simulink model "uGrid_1PH_hd_ATD2"  (R2018a)
settings: Solver=VariableStepAuto  StartTime=0.0  StopTime=0.8  FixedStep=1e-6  MaxStep=1e-4  RelTol=1e-3
PreLoadFcn:
  | SimulinkInit
InitFcn:
  | SimulinkInit
StopFcn:
  | EndingScript
values from neighbouring files (symbols this model uses):
  Ad = sysd.A    [SimulinkInit.m]
  Bd = sysd.B    [SimulinkInit.m]
  C1 = Cd(2,:)    [SimulinkInit.m]
  C10 = Cd(1,:)    [SimulinkInit.m]
  C11 = Cd(2,:)    [SimulinkInit.m]
  C12 = Cd(3,:)    [SimulinkInit.m]
  C2 = Cd(3,:)    [SimulinkInit.m]
  C3 = Cd(4,:)    [SimulinkInit.m]
  C4 = Cd(1,:)    [SimulinkInit.m]
  C5 = Cd(3,:)    [SimulinkInit.m]
  C6 = Cd(4,:)    [SimulinkInit.m]
  C7 = Cd(1,:)    [SimulinkInit.m]
  C8 = Cd(2,:)    [SimulinkInit.m]
  C9 = Cd(4,:)    [SimulinkInit.m]
  Cd = sysd.C    [SimulinkInit.m]
  T1 = 0.4    [parametros_BIO.m]
  T2 = 1    [parametros_BIO.m]
  T3 = 15    [parametros_BIO.m]
  T4 = 2.5    [parametros_BIO.m]
  T5 = 3.3    [parametros_BIO.m]
  Tao1 = 0.5    [SimulinkInit.m]
  tm = 1e-4    (= 0.0001)    [SimulinkInit.m]
undefined symbols (not defined in the file or in its folder): F1, F10, F11, F12, F2, F3, F4, F5, F6, F7, F8, F9, G, GF, H1, H10, H11, H12, H2, H3, H4, H5, H6, H7, H8, H9, Ion, K10U, K11U, K12U, K1U, K2U, K3U, K4U, K5U, K6U, K7U, K8U, K9U, Lithium, ss1, ss2, T10, T11, T12, T6, T7, T8, T9
libraries: powerlib x59, dsparch4 x17, truetime x12, powerlib_meascontrol x6, simulink x2, dspstat3 x2, dspfdesign x1, electricdrivelib x1
(part 1 of 3)
settings Model: Creator=erich  LastModifiedBy=cmparedes
settings CodeAppCC: StateflowObjectComments=on
settings SimscapeCC: SimscapeNormalizeSystem=off

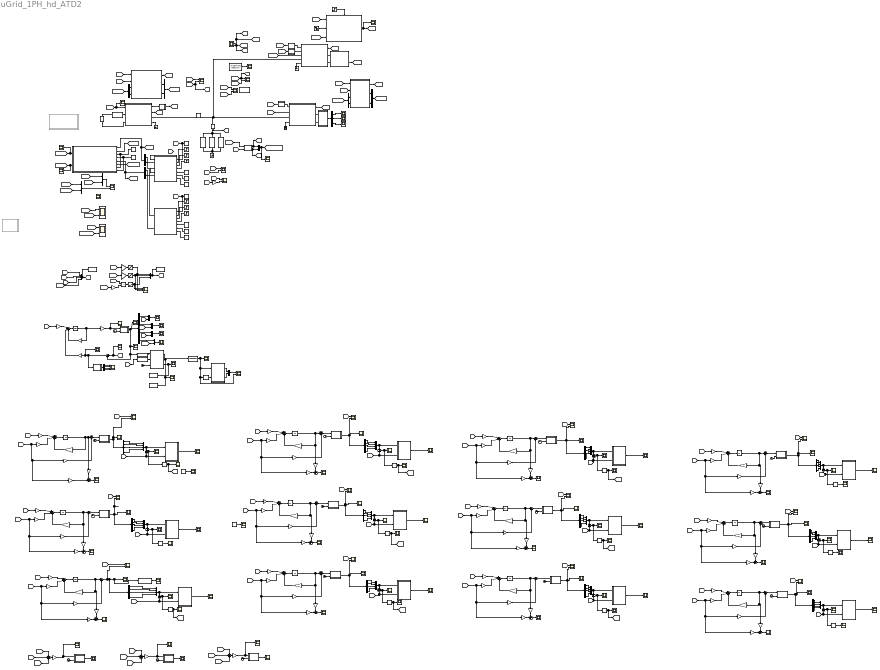
== system uGrid_1PH_hd_ATD2 ==
  note: DIESEL VSI
  note: Load
  note: BIO - CSI
  note: RENEWABLE - CSI
  note: Nodo De Optimizacion
  1Ph_Inverter_bio : Subsystem  mask{st_time=0, f_sw=12000, samp_f=1e-6}
      mask prompts: st_time "Tiempo muerto (Start)"; f_sw "Switching frequency"; samp_f "samplig"
      mask Display:
      | port_label('input', 1, 'd', 'texmode', 'on')
      | 
      | port_label('lconn', 1, 'DC +')
      | port_label('lconn', 2, 'DC -')
      | 
      | 
      | port_label('rconn', 1, 'V_{out+}')
      | port_label('rconn', 2, 'B_{out-}')
      | 
      | 
      | port_label('output', 1, 'I_{out}', 'texmode', 'on')
      | port_label('output', 2, 'V_{out}', 'texmode', 'on')
      | 
      | plot([0.1 .9], [0.1 .9])
      | plot([0.2 .4], [.7 .7])
      | plot([0.2 .24], [.65 .65])
      | plot([0.28 .32], [.65 .65])
      | plot([0.36 .40], [.65 .65])
      | 
      | plot([.5:.01:.7], .25+sin(30*[.2:.01:.4])/10)
  1Ph_Inverter_bio1 : Subsystem  mask{st_time=0, f_sw=12000, samp_f=1e-6}
      mask prompts: st_time "Tiempo muerto (Start)"; f_sw "Switching frequency"; samp_f "samplig"
      mask Display:
      | port_label('input', 1, 'd', 'texmode', 'on')
      | 
      | port_label('lconn', 1, 'DC +')
      | port_label('lconn', 2, 'DC -')
      | 
      | 
      | port_label('rconn', 1, 'V_{out+}')
      | port_label('rconn', 2, 'B_{out-}')
      | 
      | 
      | port_label('output', 1, 'I_{out}', 'texmode', 'on')
      | port_label('output', 2, 'V_{out}', 'texmode', 'on')
      | port_label('output', 3, 'I_{cap}', 'texmode', 'on')
      | 
      | plot([0.1 .9], [0.1 .9])
      | plot([0.2 .4], [.7 .7])
      | plot([0.2 .24], [.65 .65])
      | plot([0.28 .32], [.65 .65])
      | plot([0.36 .40], [.65 .65])
      | 
      | plot([.5:.01:.7], .25+sin(30*[.2:.01:.4])/10)
  1Ph_Inverter_diesel : Subsystem  mask{st_time=0, f_sw=12000, samp_f=1e-6}
      mask prompts: st_time "Tiempo muerto (Start)"; f_sw "Switching frequency"; samp_f "Sampling frequency"
      mask Display:
      | port_label('input', 1, 'd', 'texmode', 'on')
      | 
      | port_label('lconn', 1, 'DC +')
      | port_label('lconn', 2, 'DC -')
      | 
      | 
      | port_label('rconn', 1, 'V_{out+}')
      | port_label('rconn', 2, 'B_{out-}')
      | 
      | 
      | port_label('output', 1, 'I_{out}', 'texmode', 'on')
      | port_label('output', 2, 'V_{out}', 'texmode', 'on')
      | 
      | plot([0.1 .9], [0.1 .9])
      | plot([0.2 .4], [.7 .7])
      | plot([0.2 .24], [.65 .65])
      | plot([0.28 .32], [.65 .65])
      | plot([0.36 .40], [.65 .65])
      | 
      | plot([.5:.01:.7], .25+sin(30*[.2:.01:.4])/10)
  BioMassGenerator : Subsystem  Commented=on
  Bus Selector : BusSelector  OutputSignals=SOC (%),Current (A),Voltage (V)
  CSI_Control_BIO : Subsystem
  CSI_Control_DIESEL : Subsystem
  Clock{,1,3..16} (16 alike) : Clock
  Constant : Constant  Value=1000
  Constant{1,4..5,7} (4 alike) : Constant  Value=4000
  Constant2 : Constant  Value=11210
  Constant3 : Constant  Value=5000
  Constant6 : Constant  Value=5000
  DC 1000V : powerlib/Electrical Sources/DC Voltage Source  Amplitude=1000  Measurements=None
  DIESEL + Rectifier System : Subsystem
  Delay2 : Delay  DelayLength=1
  Demux : Demux  Outputs=2
  Demux1 : Demux  Outputs=2
  Demux{3..14} (12 alike) : Demux  Outputs=5
  Demux19 : Demux
  Demux2 : Demux
  Derivative{,1..2,4..12} (12 alike) : Derivative  CoefficientInTFapproximation=0
  Derivative3 : Derivative
  DynMat : Constant  Value=G
  DynMat_RespLibre : Constant  Value=GF
  FRACASO : Subsystem  Commented=on
  Gain : Gain  Gain=1/3
  Gain1 : Gain  Gain=1/3
  Gain2 : Gain  Gain=-1
  Gain3 : Gain  Gain=1/3
  Gain4 : Gain  Gain=2000
  Gain5 : Gain  Gain=2
  Gain6 : Gain  Gain=2000
  Ground{,1..3} (4 alike) : powerlib/Elements/Ground  LConnTagsString=a
  Highpass Filter : dspfdesign/Highpass Filter  FilterType=FIR  DesignForMinimumOrder=on  FilterOrder=50  StopbandFrequency=50  PassbandFrequency=60  StopbandAttenuation=80  PassbandRipple=0.1  InheritSampleRate=off  SampleRate=1/tm  SimulateUsing=Interpreted execution  roundingMode=Floor  coeffsDataTypeStr=fixdt(1,16)
      settings: SourceProductName=DSP System Toolbox
  Hw5 : dsparch4/Analog Filter Design  method=Bessel  filttype=Lowpass  N=20  Wlo=60*2*pi  Whi=80  Rp=2  Rs=80
  I sens A : powerlib/Measurements/Current Measurement  PhasorSimulation=off  OutputType=Complex  PSBequivalent=0
  LinearProg : MATLAB Function  TreatAsAtomicUnit=on  SystemSampleTime=1e-3
  LinearProg1 : MATLAB Function  TreatAsAtomicUnit=on  SystemSampleTime=1e-3
  MATLAB Function : MATLAB Function  TreatAsAtomicUnit=on
  MATLAB Function1 : MATLAB Function  TreatAsAtomicUnit=on
  MATLAB Function12 : MATLAB Function  TreatAsAtomicUnit=on
  MATLAB Function13 : MATLAB Function  TreatAsAtomicUnit=on
  MATLAB Function15 : MATLAB Function  TreatAsAtomicUnit=on
  MATLAB Function16 : MATLAB Function  TreatAsAtomicUnit=on
  MATLAB Function17 : MATLAB Function  TreatAsAtomicUnit=on
  MATLAB Function18 : MATLAB Function  TreatAsAtomicUnit=on
  MATLAB Function19 : MATLAB Function  TreatAsAtomicUnit=on
  MATLAB Function2 : MATLAB Function  TreatAsAtomicUnit=on
  MATLAB Function20 : MATLAB Function  TreatAsAtomicUnit=on
  MATLAB Function21 : MATLAB Function  TreatAsAtomicUnit=on
  MATLAB Function22 : MATLAB Function  TreatAsAtomicUnit=on
  MATLAB Function24 : MATLAB Function  TreatAsAtomicUnit=on
  MATLAB Function25 : MATLAB Function  TreatAsAtomicUnit=on
  MATLAB Function26 : MATLAB Function  TreatAsAtomicUnit=on
  MATLAB Function27 : MATLAB Function  TreatAsAtomicUnit=on
  MATLAB Function28 : MATLAB Function  TreatAsAtomicUnit=on
  MATLAB Function29 : MATLAB Function  TreatAsAtomicUnit=on
  MATLAB Function3 : MATLAB Function  TreatAsAtomicUnit=on
  MATLAB Function30 : MATLAB Function  TreatAsAtomicUnit=on
  MATLAB Function31 : MATLAB Function  TreatAsAtomicUnit=on
  MATLAB Function32 : MATLAB Function  TreatAsAtomicUnit=on
  MATLAB Function33 : MATLAB Function  TreatAsAtomicUnit=on
  MATLAB Function34 : MATLAB Function  TreatAsAtomicUnit=on
  MATLAB Function35 : MATLAB Function  TreatAsAtomicUnit=on
  MATLAB Function37 : MATLAB Function  TreatAsAtomicUnit=on
  MATLAB Function7 : MATLAB Function  TreatAsAtomicUnit=on
  MATLAB Function8 : MATLAB Function  TreatAsAtomicUnit=on
  MATLAB Function9 : MATLAB Function  TreatAsAtomicUnit=on
  MPC Controller : Subsystem
  MeasureNode_I1 : Subsystem
  MeasureNode_I2 : Subsystem
  MeasureNode_I3 : Subsystem
  MeasureNode_I4 : Subsystem
  Mux{,1..6,9..12,14} (12 alike) : Mux  Inputs=2
  Mux{8,13,15..25} (13 alike) : Mux
  Mux7 : Mux  Inputs=3
  P_lp_bio : Constant  Value=500
  P_lp_diesel : Constant  Value=300
  Power : powerlib_meascontrol/Measurements/Power  Freq=60  Vinit=[1, 0]  Iinit=[1, 0]  Ts=0
      settings: SourceProductName=Simscape Power Systems
  Product1 : Product
  RL : powerlib/Elements/Series RLC Branch  LConnTagsString=__new0  RConnTagsString=__new0  BranchType=R  Resistance=10  Inductance=500e-3  SetiL0=off  InitialCurrent=0  Capacitance=100e-6  Setx0=off  InitialVoltage=0  Measurements=None
  RL1 : powerlib/Elements/Series RLC Branch  LConnTagsString=__new0  RConnTagsString=__new0  BranchType=RL  Resistance=10  Inductance=5.2  SetiL0=off  InitialCurrent=0  Capacitance=100e-6  Setx0=off  InitialVoltage=0  Measurements=None
  RL2 : powerlib/Elements/Series RLC Branch  LConnTagsString=__new0  RConnTagsString=__new0  BranchType=C  Resistance=30  Inductance=500e-3  SetiL0=off  InitialCurrent=0  Capacitance=2000e-6  Setx0=off  InitialVoltage=0  Measurements=None
  Rin : powerlib/Elements/Series RLC Branch  LConnTagsString=__new0  RConnTagsString=__new0  BranchType=R  Resistance=.001  Inductance=0  SetiL0=off  InitialCurrent=0  Capacitance=0  Setx0=off  InitialVoltage=0  Measurements=None
  Saturation3 : Saturate  UpperLimit=1000  LowerLimit=-1000
  Saturation4 : Saturate  UpperLimit=1000  LowerLimit=-1000
  Saturation5 : Saturate  UpperLimit=1000  LowerLimit=-1000
  Scope{,1..3,7,24..25,27..28,42,85..95,97} (22 alike) : Scope  NumInputPorts=2
  Scope{4..6,8..17,19..23,26,29,31..41,44,46..60,63..84,96,98,100..119} (91 alike) : Scope
  Scope30 : Scope  NumInputPorts=3
  Scope43 : Scope  NumInputPorts=4
  Signal Specification : SignalSpecification  Dimensions=4
  Signal Specification1 : SignalSpecification  Dimensions=4
  Sine Wave : Sin  Amplitude=170  Frequency=2*pi*60  SampleTime=0
  Step1 : Step  Time=0.3  Before=20000  After=5000  SampleTime=0
  Step2 : Step  Time=.6  Before=1.2  After=.4  SampleTime=0
  Step3 : Step  Before=.7  After=.7  SampleTime=0
  Step4 : Step  Time=10e-3  SampleTime=0
  Step5 : Step  Time=.3  Before=20000  After=5000  SampleTime=0
  Step6 : Step  Time=.6  Before=1.2  After=.4  SampleTime=0
  Step7 : Step  Before=.7  After=.7  SampleTime=0
  Subsystem : Subsystem
  Sum{,3,7,15,18,22,30,34,36,42,46,48} (12 alike) : Sum  Inputs=|++
  Sum{1..2,5,11,13,20,26,28,32,38,40,44} (12 alike) : Sum  Inputs=+-
  Sum10 : Sum  Inputs=|+-
  Sum{6,12,17,21,23..24,27,29,33,39,41,45} (12 alike) : Sum  Inputs=-+|
  Sum{4,8..9,14,16,19,25,31,35,37,43,47,49} (13 alike) : Sum  Inputs=|+++  SampleTime=tm
  Sum50 : Sum  Inputs=+++
  Sum51 : Sum  Inputs=+++
  Sum52 : Sum  Inputs=+++
  To Workspace : ToWorkspace  VariableName=det1  SampleTime=1e-4
  To Workspace1 : ToWorkspace  VariableName=norm1  SampleTime=1e-4
  To Workspace2 : ToWorkspace  VariableName=y_ma  SampleTime=1e-4
  To Workspace3 : ToWorkspace  VariableName=u_fs  SampleTime=1e-4
  Transfer Fcn6 : TransferFcn  Denominator=[0.005 1]
  TrueTime Network : truetime/TrueTime Network  nwtype=CSMA/CD (Ethernet)  nwnbr=1  nnodes=10  rate=8*1e9  minsize=512  lossprob=0  seed=0  bandwidths=[0.5 0.5]  slotsize=512  schedule=[1 1 2]  memsize=80000  buftype=Common buffer  overflow=Retransmit  dynSchedule=0  miniSlotSize=0  NIT=0  QSortMode=FIFO  sync=0  irtSchedule=0  nrtLength=0  nodeGraph=0  scheduleoutput=on
  Unit Delay{1..13} (13 alike) : UnitDelay  SampleTime=tm
  VSI_Controller : Subsystem
  adis1 : Gain  Gain=F3  Multiplication=Matrix(K*u) (u vector)  SampleTime=tm
  adis10 : Gain  Gain=Ld'  Multiplication=Matrix(K*u) (u vector)  SampleTime=tm
  adis11 : Gain  Gain=F1  Multiplication=Matrix(K*u) (u vector)  SampleTime=tm
  adis12 : Gain  Gain=F2  Multiplication=Matrix(K*u) (u vector)  SampleTime=tm
  adis13 : Gain  Gain=F11  Multiplication=Matrix(K*u) (u vector)  SampleTime=tm
  adis14 : Gain  Gain=F12  Multiplication=Matrix(K*u) (u vector)  SampleTime=tm
  adis2 : Gain  Gain=F4  Multiplication=Matrix(K*u) (u vector)  SampleTime=tm
  adis3 : Gain  Gain=F5  Multiplication=Matrix(K*u) (u vector)  SampleTime=tm
  adis4 : Gain  Gain=F6  Multiplication=Matrix(K*u) (u vector)  SampleTime=tm
  adis5 : Gain  Gain=F7  Multiplication=Matrix(K*u) (u vector)  SampleTime=tm
  adis6 : Gain  Gain=F8  Multiplication=Matrix(K*u) (u vector)  SampleTime=tm
  adis7 : Gain  Gain=Ad  Multiplication=Matrix(K*u) (u vector)  SampleTime=tm
  adis8 : Gain  Gain=F9  Multiplication=Matrix(K*u) (u vector)  SampleTime=tm
  adis9 : Gain  Gain=F10  Multiplication=Matrix(K*u) (u vector)  SampleTime=tm
  bdis1 : Gain  Gain=T3*Bd  Multiplication=Matrix(K*u) (u vector)  SampleTime=tm
  bdis10 : Gain  Gain=T2*Bd  Multiplication=Matrix(K*u) (u vector)  SampleTime=tm
  bdis11 : Gain  Gain=K2U  Multiplication=Matrix(K*u) (u vector)  SampleTime=tm
  bdis12 : Gain  Gain=H2  Multiplication=Matrix(K*u) (u vector)  SampleTime=tm
  bdis13 : Gain  Gain=eye(1)-C2*H2  Multiplication=Matrix(K*u) (u vector)  SampleTime=tm
  bdis14 : Gain  Gain=eye(1)-C1*H1  Multiplication=Matrix(K*u) (u vector)  SampleTime=tm
  bdis15 : Gain  Gain=C1  Multiplication=Matrix(K*u) (u vector)  SampleTime=tm
  bdis16 : Gain  Gain=C2  Multiplication=Matrix(K*u) (u vector)  SampleTime=tm
  bdis17 : Gain  Gain=T4*Bd  Multiplication=Matrix(K*u) (u vector)  SampleTime=tm
  bdis18 : Gain  Gain=K4U  Multiplication=Matrix(K*u) (u vector)  SampleTime=tm
  bdis19 : Gain  Gain=H4  Multiplication=Matrix(K*u) (u vector)  SampleTime=tm
  bdis2 : Gain  Gain=K3U  Multiplication=Matrix(K*u) (u vector)  SampleTime=tm
  bdis20 : Gain  Gain=eye(1)-C4*H4  Multiplication=Matrix(K*u) (u vector)  SampleTime=tm
  bdis21 : Gain  Gain=C4  Multiplication=Matrix(K*u) (u vector)  SampleTime=tm
  bdis22 : Gain  Gain=T5*Bd  Multiplication=Matrix(K*u) (u vector)  SampleTime=tm
  bdis23 : Gain  Gain=K5U  Multiplication=Matrix(K*u) (u vector)  SampleTime=tm
  bdis24 : Gain  Gain=H5  Multiplication=Matrix(K*u) (u vector)  SampleTime=tm
  bdis25 : Gain  Gain=eye(1)-C5*H5  Multiplication=Matrix(K*u) (u vector)  SampleTime=tm
  bdis26 : Gain  Gain=C5  Multiplication=Matrix(K*u) (u vector)  SampleTime=tm
  bdis27 : Gain  Gain=T6*Bd  Multiplication=Matrix(K*u) (u vector)  SampleTime=tm
  bdis28 : Gain  Gain=K6U  Multiplication=Matrix(K*u) (u vector)  SampleTime=tm
  bdis29 : Gain  Gain=H6  Multiplication=Matrix(K*u) (u vector)  SampleTime=tm
  bdis3 : Gain  Gain=H3  Multiplication=Matrix(K*u) (u vector)  SampleTime=tm
  bdis30 : Gain  Gain=eye(1)-C6*H6  Multiplication=Matrix(K*u) (u vector)  SampleTime=tm
  bdis31 : Gain  Gain=C6  Multiplication=Matrix(K*u) (u vector)  SampleTime=tm
  bdis32 : Gain  Gain=T7*Bd  Multiplication=Matrix(K*u) (u vector)  SampleTime=tm
  bdis33 : Gain  Gain=K7U  Multiplication=Matrix(K*u) (u vector)  SampleTime=tm
  bdis34 : Gain  Gain=H7  Multiplication=Matrix(K*u) (u vector)  SampleTime=tm
  bdis35 : Gain  Gain=eye(1)-C7*H7  Multiplication=Matrix(K*u) (u vector)  SampleTime=tm
  bdis36 : Gain  Gain=C7  Multiplication=Matrix(K*u) (u vector)  SampleTime=tm
  bdis37 : Gain  Gain=T8*Bd  Multiplication=Matrix(K*u) (u vector)  SampleTime=tm
  bdis38 : Gain  Gain=K8U  Multiplication=Matrix(K*u) (u vector)  SampleTime=tm
  bdis39 : Gain  Gain=H8  Multiplication=Matrix(K*u) (u vector)  SampleTime=tm
  bdis4 : Gain  Gain=eye(1)-C3*H3  Multiplication=Matrix(K*u) (u vector)  SampleTime=tm
  bdis40 : Gain  Gain=eye(1)-C8*H8  Multiplication=Matrix(K*u) (u vector)  SampleTime=tm
  bdis41 : Gain  Gain=C8  Multiplication=Matrix(K*u) (u vector)  SampleTime=tm
  bdis42 : Gain  Gain=T9*Bd  Multiplication=Matrix(K*u) (u vector)  SampleTime=tm
  bdis43 : Gain  Gain=K9U  Multiplication=Matrix(K*u) (u vector)  SampleTime=tm
  bdis44 : Gain  Gain=H9  Multiplication=Matrix(K*u) (u vector)  SampleTime=tm
  bdis45 : Gain  Gain=eye(1)-C9*H9  Multiplication=Matrix(K*u) (u vector)  SampleTime=tm
  bdis46 : Gain  Gain=C9  Multiplication=Matrix(K*u) (u vector)  SampleTime=tm
  bdis47 : Gain  Gain=T10*Bd  Multiplication=Matrix(K*u) (u vector)  SampleTime=tm
  bdis48 : Gain  Gain=K10U  Multiplication=Matrix(K*u) (u vector)  SampleTime=tm
  bdis49 : Gain  Gain=H10  Multiplication=Matrix(K*u) (u vector)  SampleTime=tm
  bdis5 : Gain  Gain=Bd  Multiplication=Matrix(K*u) (u vector)  SampleTime=tm
  bdis50 : Gain  Gain=eye(1)-C10*H10  Multiplication=Matrix(K*u) (u vector)  SampleTime=tm
  bdis51 : Gain  Gain=C10  Multiplication=Matrix(K*u) (u vector)  SampleTime=tm
  bdis52 : Gain  Gain=T11*Bd  Multiplication=Matrix(K*u) (u vector)  SampleTime=tm
  bdis53 : Gain  Gain=K11U  Multiplication=Matrix(K*u) (u vector)  SampleTime=tm
  bdis54 : Gain  Gain=H11  Multiplication=Matrix(K*u) (u vector)  SampleTime=tm
  bdis55 : Gain  Gain=eye(1)-C11*H11  Multiplication=Matrix(K*u) (u vector)  SampleTime=tm
  bdis56 : Gain  Gain=C11  Multiplication=Matrix(K*u) (u vector)  SampleTime=tm
  bdis57 : Gain  Gain=T12*Bd  Multiplication=Matrix(K*u) (u vector)  SampleTime=tm
  bdis58 : Gain  Gain=K12U  Multiplication=Matrix(K*u) (u vector)  SampleTime=tm
  bdis59 : Gain  Gain=H12  Multiplication=Matrix(K*u) (u vector)  SampleTime=tm
  bdis6 : Gain  Gain=C3  Multiplication=Matrix(K*u) (u vector)  SampleTime=tm
  bdis60 : Gain  Gain=eye(1)-C12*H12  Multiplication=Matrix(K*u) (u vector)  SampleTime=tm
  bdis61 : Gain  Gain=C12  Multiplication=Matrix(K*u) (u vector)  SampleTime=tm
  bdis7 : Gain  Gain=T1*Bd  Multiplication=Matrix(K*u) (u vector)  SampleTime=tm
  bdis8 : Gain  Gain=K1U  Multiplication=Matrix(K*u) (u vector)  SampleTime=tm
  bdis9 : Gain  Gain=H1  Multiplication=Matrix(K*u) (u vector)  SampleTime=tm
  cdis4 : Gain  Gain=Cd  Multiplication=Matrix(K*u) (u vector)  SampleTime=tm
  powergui : powerlib/powergui  Priority=1  SimulationMode=Continuous  SampleTime=50e-6  frequency=60  Iterations=50  frequencyindice=0  Pbase=100e6  ErrMax=1e-4  UnitsV=kV  UnitsW=MW  buscounter=0  FunctionMessages=off  echomessages=off  EnableUseOfTLC=off  CurrentSourceSwitches=off  DisableSnubberDevices=off  DisableRonSwitches=off  DisableVfSwitches=off  DisplayEquations=off  SolverType=Tustin/Backward Euler (TBE)  Interpol=off  ExternalGateDelay=off  methode=off  Ts=100  x0status=blocks  SPID=on  SwTol=0  HookPort=off  RestoreLinks=warning  ResistiveCurrentMeasurement=off  Frange=[0:2:500]  Ylog=off  Xlog=on  ShowGrid=off  save=off  variable=ZData  structure=0  ZoomFFT=off  StartTime=0.0  cycles=1  DisplayStyle=1  fundamental=60  FreqAxis=off  MaxFrequency=1000  frequencyindicesteady=1  RmsSteady=1  display=off
  1000 : Constant  IOType=siggen
  wires:
  [D_bio] -> Scope4/1, 1Ph_Inverter_bio/1(A_in)
  [D_die] -> 1Ph_Inverter_diesel/1(A_in)
  [I_bio] -> [I1], Scope2/2
  [V_bio] -> Scope2/1
  [I_die] -> [I2], Scope3/1
  [V_die] -> Scope3/2
  1Ph_Inverter_bio/1(Iout) -> MeasureNode_I2/1(in)
  1Ph_Inverter_bio/2(Vout) -> [V_bio]
  1Ph_Inverter_diesel/1(Iout) -> MeasureNode_I1/1(in)
  1Ph_Inverter_diesel/2(Vout) -> [V_die]
  CSI_Control_BIO/1(D) -> [D_bio]
  [I_bio] -> CSI_Control_BIO/2(I_measured)
  [V_bio] -> CSI_Control_BIO/1(V_measured)
  CSI_Control_DIESEL/1(D) -> [D_die]
  [I_die] -> CSI_Control_DIESEL/2(I_measured)
  [V_die] -> CSI_Control_DIESEL/1(V_measured)
  [I_vsi] -> Scope1/1
  [I_load] -> Scope1/2
  Mux/1 -> [PQ_meas_bio]
  [MPC_U_bio] -> Demux/1
  [MPC_U_diesel] -> Demux1/1
  Mux1/1 -> [PQ_meas_diesel]
  [set_DIESEL] -> Mux2/2  "set_DIESEL"
  [set_BIO] -> Mux2/1  "set_BIO"
  Mux2/1 -> Scope/1
  Mux3/1 -> Scope/2
  [PQ_meas_diesel] -> Mux3/2  "meas_DIESEL"
  [PQ_meas_bio] -> Mux3/1  "meas_BIO"
  CSI_Control_BIO/2(P_measure) -> Mux/1
  CSI_Control_BIO/3(Q_measure) -> Mux/2
  CSI_Control_DIESEL/2(P_measure) -> Mux1/1
  CSI_Control_DIESEL/3(Q_measure) -> Mux1/2
  Demux1/1 -> CSI_Control_DIESEL/3(P_ref)
  Demux1/2 -> CSI_Control_DIESEL/4(Q_ref)
  Demux/1 -> CSI_Control_BIO/3(P_ref)
  Demux/2 -> CSI_Control_BIO/4(Q_ref)
  DynMat_RespLibre/1 -> MPC Controller/4(GF_bio), MPC Controller/8(GF_Diesel)
  DynMat/1 -> MPC Controller/3(G_bio), MPC Controller/7(G_Diesel)
  MPC Controller/2(MPC_DIESEL_OUT) -> [MPC_U_diesel], Scope9/1
  MPC Controller/1(MPC_BIO_OUT) -> Scope5/1, [MPC_U_bio]
  [PQ_meas_bio] -> MPC Controller/2(PQ_meas_bio)
  [PQ_meas_diesel] -> MPC Controller/6(PQ_meas_Diesel)
  Constant3/1 -> LinearProg/7(P_e_alt_min)
  Constant5/1 -> LinearProg/6(PbMax)
  Step2/1 -> LinearProg/3(kb)
  Step3/1 -> LinearProg/4(kd)
  Constant1/1 -> LinearProg/5(PdMax)
  Step1/1 -> LinearProg/2(P_e_alt)
  Mux5/1 -> [set_DIESEL], MPC Controller/5(PQref_Diesel)
  Mux4/1 -> MPC Controller/1(PQref_Bio), [set_BIO]
  VSI_Controller/1(d) -> Scope6/1, [D_vsi]
  [I_vsi] -> VSI_Controller/1(Output Current)  "OutputCurrent"
  Sine Wave/1 -> VSI_Controller/2(Ref Voltage)  "Vc_ref"
  [I_cap_vsi] -> VSI_Controller/3(Capacitor Current)
  1Ph_Inverter_bio1/3(I cap) -> [I_cap_vsi]
  [D_vsi] -> 1Ph_Inverter_bio1/1(A_in)
  1Ph_Inverter_bio1/2(Vout) -> MeasureNode_I3/1(in)
  [V_vsi] -> Scope7/1, [Vlreal]  "v load"
  [I_vsi] -> [I3], Scope7/2
  MeasureNode_I2/1(Out) -> [I_bio]
  MeasureNode_I1/1(Out) -> [I_die]
  MeasureNode_I4/1(Out) -> [I_vsi]
  1Ph_Inverter_bio1/1(Iout) -> MeasureNode_I4/1(in)
  I sens A/1 -> [I_load]
  MeasureNode_I3/1(Out) -> [V_vsi]
  DIESEL + Rectifier System/2(Output DC Voltage) -> [DieselE]
  Bus Selector/2 -> Scope10/1  "<Current (A)>"
  Bus Selector/1 -> Scope12/1  "<SOC (%)>"
  Bus Selector/3 -> Scope11/1  "<Voltage (V)>"
  Subsystem/1(Out1) -> Bus Selector/1
  Step4/1 -> VSI_Controller/Enable
  TrueTime Network/1 -> Scope13/1
  Power/2 -> [Q_load], Mux6/2
  [I_load] -> Power/2
  Mux6/1 -> Scope23/1, [Potencia_Meas]
  [V_vsi] -> Power/1  "v load"
  Power/1 -> [P_load], Mux6/1
  Constant4/1 -> LinearProg1/5(QdMax)
  Step5/1 -> LinearProg1/2(Q_e_alt)
  Constant7/1 -> LinearProg1/6(QbMax)
  Step6/1 -> LinearProg1/3(kb)
  Step7/1 -> LinearProg1/4(kd)
  Constant6/1 -> LinearProg1/7(Q_e_alt_min)
  LinearProg/1(Pbo) -> Mux4/1  "bio"
  LinearProg/2(Pdo) -> Mux5/1  "die"
  LinearProg1/1(Qbo) -> Mux4/2
  LinearProg1/2(Qdo) -> Mux5/2
  [set_BIO] -> Scope24/1
  [PQ_meas_bio] -> Scope24/2
  [set_DIESEL] -> Scope25/1
  [PQ_meas_diesel] -> Scope25/2
  Constant/1 -> [P_ref], LinearProg/1(P_load)
  Constant2/1 -> [Q_ref], LinearProg1/1(Q_load)
  [P_load] -> Scope27/1
  [P_ref] -> Scope27/2
  [Q_load] -> Scope28/1
  [Q_ref] -> Gain2/1
  Gain2/1 -> Scope28/2
  Product1/1 -> Saturation5/1
  Gain5/1 -> Product1/2
  Saturation3/1 -> Scope30/3, Mux7/1
  Gain6/1 -> Saturation4/1
  [D_die] -> Gain6/1
  [DieselE] -> Gain5/1
  [D_vsi] -> Product1/1
  Saturation5/1 -> Mux7/3, Scope30/1
  Gain4/1 -> Saturation3/1
  Saturation4/1 -> Scope30/2, Mux7/2
  [D_bio] -> Gain4/1
  Mux7/1 -> To Workspace3/1, [u_fs]
  [V_vsi] -> Mux8/4
  Mux8/1 -> To Workspace2/1, [y_ma]
  [I1] -> Mux8/1
  [I2] -> Mux8/2
  [I3] -> Mux8/3
  Demux19/4 -> Scope43/4
  MATLAB Function3/1(rol) -> To Workspace/1, Scope36/1, Transfer Fcn6/1
  MATLAB Function7/2(Th_det) -> Mux14/2
  cdis4/1 -> MATLAB Function1/1(y_hat), Scope35/1
  Delay2/1 -> MATLAB Function7/2(r1)
  [y_ma] -> Signal Specification1/1
  adis10/1 -> Sum8/2
  [y_ma] -> Scope33/1, Sum10/1
  Mux14/1 -> Scope42/1
  Unit Delay6/1 -> cdis4/1, adis7/1
  [I2] -> Mux10/2
  Demux19/2 -> Scope43/2
  Sum10/1 -> MATLAB Function2/1(r), Scope37/1, adis10/1
  MATLAB Function2/1(y) -> Demux19/1
  Mux9/1 -> Scope31/1
  Demux2/1 -> Mux9/1
  [I3] -> Mux11/2
  Mux12/1 -> Scope34/1
  Mux11/1 -> Scope38/1
  Demux2/3 -> Mux11/1
  Clock1/1 -> MATLAB Function3/3(tiempo)
  MATLAB Function1/1(y) -> Scope8/1, Demux2/1, Scope40/1, Sum10/2, Signal Specification/1
  Mux10/1 -> Scope32/1
  MATLAB Function7/1(rol) -> Mux14/1
  [u_fs] -> bdis5/1
  Signal Specification/1 -> MATLAB Function3/1(y_hat)
  bdis5/1 -> Sum8/1
  Demux19/3 -> Scope43/3
  Transfer Fcn6/1 -> Scope42/2, Delay2/1, MATLAB Function7/1(r), Scope41/1
  [I1] -> Mux9/2
  Sum8/1 -> Unit Delay6/1
  Demux2/2 -> Mux10/1
  Demux2/4 -> Mux12/1
  Clock/1 -> MATLAB Function1/2(t)
  MATLAB Function3/2(norm_rd) -> To Workspace1/1, Scope39/1
  Signal Specification1/1 -> MATLAB Function3/2(y_m)
  adis7/1 -> Sum8/3
  [V_vsi] -> Mux12/2
  Demux19/1 -> Scope43/1
  Clock16/1 -> MATLAB Function35/2(t)
  [I1] -> bdis20/1, bdis19/1, bdis18/1
  Sum37/1 -> Unit Delay5/1
  Sum52/1 -> Gain3/1
  bdis55/1 -> Sum41/2
  bdis20/1 -> Sum12/2
  Demux5/1 -> Mux16/1
  Demux3/2 -> Mux13/2
  MATLAB Function18/1(ruo4) -> Scope46/1
  Clock8/1 -> MATLAB Function28/2(t)
  Sum42/1 -> MATLAB Function33/1(u)
  Derivative11/1 -> Scope103/1
  MATLAB Function32/1(y) -> Demux12/1, Scope97/2, Scope84/1
  bdis61/1 -> Sum45/1
  Derivative5/1 -> [druo5], Scope116/1
  Derivative4/1 -> [druo4], Scope115/1
  Gain3/1 -> MATLAB Function35/1(dr), Scope112/1
  Sum49/1 -> Unit Delay11/1
  [y_ma] -> Scope93/1
  [y_ma] -> Scope94/1
  MATLAB Function19/1(ruo4) -> Scope19/1
  Demux5/2 -> Mux16/2
  Mux18/1 -> Sum5/1, MATLAB Function12/1(ya)
  Demux10/3 -> Mux23/3
  [y_ma] -> Scope91/1
  [y_ma] -> Scope92/1
  Demux12/2 -> Mux20/2
  Unit Delay13/1 -> bdis61/1, adis14/1, Sum46/1
  [y_ma] -> Scope89/1
  adis6/1 -> Sum31/3
  Demux13/5 -> Mux15/4
  Demux6/2 -> Mux17/2
  Demux10/2 -> Mux23/2
  Demux11/1 -> Mux25/1
  MATLAB Function35/1(r) -> Scope109/1
  bdis16/1 -> Sum24/1
  [y_ma] -> Sum44/2, MATLAB Function22/2(ym)
  Demux13/2 -> Mux15/2
  Clock4/1 -> MATLAB Function24/2(t)
  Sum40/1 -> Derivative11/1, Scope77/1
  bdis43/1 -> Sum35/2
  adis13/1 -> Sum43/3
  MATLAB Function27/1(y) -> Demux4/1, Scope90/2, Scope96/1
  [y_ma] -> Sum40/2, MATLAB Function21/2(ym)
  Sum43/1 -> Unit Delay12/1
  bdis29/1 -> Sum22/2
  bdis38/1 -> Sum31/2
  Sum38/1 -> Derivative10/1, Scope79/1
  [y_ma] -> Sum13/2, MATLAB Function15/2(ym)
  adis9/1 -> Sum49/3
  [u_fs] -> bdis47/1
  [I1] -> bdis35/1, bdis34/1, bdis33/1
  bdis39/1 -> Sum30/2
  Demux12/3 -> Mux20/3
  bdis13/1 -> Sum24/2
  Demux3/5 -> Mux13/4
  bdis54/1 -> Sum42/2
  [y_ma] -> Scope86/1
  bdis50/1 -> Sum39/2
  Demux5/5 -> Mux16/4
  Demux12/1 -> Mux20/1
  Unit Delay12/1 -> bdis56/1, adis13/1, Sum42/1
  Sum44/1 -> Derivative12/1, Scope72/1
  Sum35/1 -> Unit Delay9/1
  Mux24/1 -> Sum32/1, MATLAB Function19/1(ya)
  Demux9/3 -> Mux22/3
  bdis24/1 -> Sum18/2
  [I2] -> bdis40/1, bdis39/1, bdis38/1
  adis2/1 -> Sum9/3
  Demux4/2 -> Mux21/2
  bdis41/1 -> Sum29/1
  Demux9/5 -> Mux22/4
  adis8/1 -> Sum35/3
  Demux7/1 -> Mux18/1
  bdis35/1 -> Sum27/2
  Sum27/1 -> Scope69/1
  bdis40/1 -> Sum29/2
  [y_ma] -> Sum26/2, MATLAB Function17/2(ym)
  [u_fs] -> bdis42/1
  [y_ma] -> Sum32/2, MATLAB Function19/2(ym)
  Demux8/1 -> Mux19/1
  bdis37/1 -> Sum31/1
  bdis46/1 -> Sum33/1
  adis5/1 -> Sum37/3
  Demux4/3 -> Mux21/3
  bdis22/1 -> Sum19/1
  MATLAB Function8/1(ruo1) -> Scope59/1
  Demux4/1 -> Mux21/1
  [I3] -> bdis60/1, bdis59/1, bdis58/1
  bdis2/1 -> Sum4/2
  bdis44/1 -> Sum34/2
  bdis32/1 -> Sum37/1
  [u_fs] -> bdis27/1
  bdis23/1 -> Sum19/2
  Sum17/1 -> Scope76/1
  bdis25/1 -> Sum17/2
  Sum20/1 -> Derivative6/1, Scope14/1
  adis3/1 -> Sum19/3
  Mux20/1 -> Sum44/1, MATLAB Function22/1(ya)
  adis4/1 -> Sum25/3
  Sum19/1 -> Unit Delay3/1
  MATLAB Function16/1(ruo4) -> Scope15/1
  Mux13/1 -> Sum13/1, MATLAB Function15/1(ya)
  Sum6/1 -> Scope60/1
  bdis49/1 -> Sum48/2
  bdis14/1 -> Sum23/2
  [y_ma] -> Scope88/1
  Sum41/1 -> Scope83/1
  [y_ma] -> Sum5/2, MATLAB Function12/2(ym)
  Sum13/1 -> Derivative5/1, Scope54/1
  [I2] -> bdis14/1, bdis9/1, bdis8/1
  Sum3/1 -> Demux7/1, Highpass Filter/1, Scope53/1, Scope87/2
  Demux6/5 -> Mux17/4
  Mux16/1 -> Sum1/1, MATLAB Function8/1(ya)
  Demux7/5 -> Mux18/4
  bdis1/1 -> Sum4/1
  bdis4/1 -> Sum6/2
  [u_fs] -> bdis17/1
  [I1] -> bdis50/1, bdis49/1, bdis48/1
  Sum2/1 -> Derivative1/1, Scope50/1
  bdis57/1 -> Sum47/1
  MATLAB Function13/1(ruo4) -> Scope66/1
  adis14/1 -> Sum47/3
  Mux21/1 -> Sum20/1, MATLAB Function16/1(ya)
  [y_ma] -> Sum28/2, MATLAB Function18/2(ym)
  Demux6/3 -> Mux17/3
  [druo9] -> Sum52/3
  bdis21/1 -> Sum12/1
  Sum12/1 -> Scope67/1
  bdis7/1 -> Sum14/1
  Unit Delay7/1 -> adis11/1, bdis15/1, Sum/1
  bdis19/1 -> Sum7/2
  Demux8/2 -> Mux19/2
  Sum4/1 -> Unit Delay1/1
  adis1/1 -> Sum4/3
  bdis17/1 -> Sum9/1
  bdis12/1 -> Sum15/2
  Demux8/5 -> Mux19/4
  [u_fs] -> bdis10/1
  bdis15/1 -> Sum23/1
  bdis11/1 -> Sum16/2
  [I3] -> bdis13/1, bdis12/1, bdis11/1
  MATLAB Function20/1(ruo4) -> Scope81/1
  adis11/1 -> Sum14/3
  bdis3/1 -> Sum3/2
  Derivative2/1 -> [druo3], Scope113/1
  Sum5/1 -> Derivative2/1, Scope55/1
  Unit Delay8/1 -> bdis41/1, adis6/1, Sum30/1
  bdis33/1 -> Sum37/2
  Sum33/1 -> Scope20/1
  Demux14/1 -> Mux24/1
  Demux11/3 -> Mux25/3
  Demux11/2 -> Mux25/2
  [druo8] -> Sum52/2
  adis12/1 -> Sum16/3
  MATLAB Function31/1(y) -> Scope94/2, Scope78/1, Demux13/1
  Sum/1 -> MATLAB Function/1(u)
  [u_fs] -> bdis1/1
  Gain1/1 -> MATLAB Function34/1(dr), Scope110/1
  [druo7] -> Sum52/1
  Sum39/1 -> Scope82/1
  Sum46/1 -> MATLAB Function32/1(u)
  Sum9/1 -> Unit Delay2/1
  [V_vsi] -> bdis45/1, bdis44/1, bdis43/1
  bdis42/1 -> Sum35/1
  [druo4] -> Sum51/1
  Unit Delay1/1 -> bdis6/1, adis1/1, Sum3/1
  Demux6/1 -> Mux17/1
  Derivative3/1 -> Scope114/1
  bdis36/1 -> Sum27/1
  bdis28/1 -> Sum25/2
  bdis34/1 -> Sum36/2
  Unit Delay3/1 -> bdis26/1, adis3/1, Sum18/1
  Unit Delay11/1 -> bdis51/1, adis9/1, Sum48/1
  Sum31/1 -> Unit Delay8/1
  Demux4/5 -> Mux21/4
  bdis27/1 -> Sum25/1
  [u_fs] -> bdis52/1
  MATLAB Function24/1(y) -> Demux6/1, Scope86/2, Scope48/1
  bdis60/1 -> Sum45/2
  Sum22/1 -> MATLAB Function27/1(u)
  bdis31/1 -> Sum21/1
  Derivative6/1 -> [druo6], Scope117/1
  Sum26/1 -> Derivative7/1, Scope44/1
  bdis18/1 -> Sum9/2
  Hw5/1 -> Scope105/1
  Gain/1 -> MATLAB Function37/1(dr), Scope108/1
  Sum11/1 -> Derivative4/1, Scope64/1
  MATLAB Function21/1(ruo4) -> Scope80/1
  [y_ma] -> Scope87/1
  bdis45/1 -> Sum33/2
  [druo2] -> Sum50/2
  MATLAB Function15/1(ruo4) -> Scope65/1
  Mux19/1 -> Sum11/1, MATLAB Function13/1(ya)
  MATLAB Function22/1(ruo4) -> Scope73/1
  Sum23/1 -> Scope57/1
  Sum30/1 -> MATLAB Function29/1(u)
  bdis6/1 -> Sum6/1
  Sum50/1 -> Gain/1
  Sum1/1 -> Derivative/1, Scope49/1
  Sum48/1 -> MATLAB Function31/1(u)
  [druo1] -> Sum50/1
  MATLAB Function12/1(ruo3) -> Scope56/1
  Demux9/1 -> Mux22/1
  [u_fs] -> bdis7/1
  [I2] -> bdis55/1, bdis54/1, bdis53/1
  MATLAB Function17/1(ruo4) -> Scope68/1
  bdis26/1 -> Sum17/1
  [y_ma] -> Scope95/1
  Demux14/5 -> Mux24/4
  Derivative/1 -> [druo1], Scope106/1
  bdis52/1 -> Sum43/1
  Demux11/5 -> Mux25/4
  MATLAB Function33/1(y) -> Demux11/1, Scope95/2, Scope75/1
  Mux22/1 -> Sum28/1, MATLAB Function18/1(ya)
  [y_ma] -> Sum2/2, MATLAB Function9/2(ym)
  Sum7/1 -> MATLAB Function25/1(u)
  Derivative9/1 -> [druo9], Scope101/1
  [druo5] -> Sum51/2
  Demux10/1 -> Mux23/1
  Sum29/1 -> Scope70/1
  [u_fs] -> bdis22/1
  Unit Delay10/1 -> bdis16/1, adis12/1, Sum15/1
  Demux14/2 -> Mux24/2
  Sum25/1 -> Unit Delay4/1
  Mux15/1 -> Sum38/1, MATLAB Function20/1(ya)
  Demux9/2 -> Mux22/2
  Sum32/1 -> Derivative9/1, Scope17/1
  [u_fs] -> bdis32/1
  Clock13/1 -> MATLAB Function33/2(t)
  Unit Delay4/1 -> bdis31/1, adis4/1, Sum22/1
  Unit Delay5/1 -> bdis36/1, adis5/1, Sum36/1
  [y_ma] -> Sum20/2, MATLAB Function16/2(ym)
  MATLAB Function9/1(ruo2) -> Scope52/1
  Derivative8/1 -> [druo8], Scope100/1
  Sum36/1 -> MATLAB Function28/1(u)
  bdis58/1 -> Sum47/2
  bdis30/1 -> Sum21/2
  Derivative10/1 -> Scope102/1
  Clock12/1 -> MATLAB Function32/2(t)
  [druo6] -> Sum51/3
  [druo3] -> Sum50/3
  Demux12/5 -> Mux20/4
  Derivative1/1 -> Scope111/1
  Sum24/1 -> Scope58/1
  Clock11/1 -> MATLAB Function31/2(t)
  Derivative7/1 -> [druo7], Scope119/1
  Sum51/1 -> Gain1/1
  bdis47/1 -> Sum49/1
  MATLAB Function37/1(r) -> Scope118/1
  Clock7/1 -> MATLAB Function27/2(t)
  Mux17/1 -> Sum2/1, MATLAB Function9/1(ya)
  Clock9/1 -> MATLAB Function29/2(t)
  MATLAB Function28/1(y) -> Demux10/1, Scope91/2, Scope26/1
  Derivative12/1 -> Scope104/1
  bdis56/1 -> Sum41/1
  Sum16/1 -> Unit Delay10/1
  bdis48/1 -> Sum49/2
  Demux3/1 -> Mux13/1
  Sum18/1 -> MATLAB Function26/1(u)
  Sum34/1 -> MATLAB Function30/1(u)
  bdis9/1 -> Sum/2
  [y_ma] -> Sum38/2, MATLAB Function20/2(ym)
  bdis59/1 -> Sum46/2
  MATLAB Function26/1(y) -> Scope47/1, Scope89/2, Demux3/1
  Clock10/1 -> MATLAB Function30/2(t)
  Sum47/1 -> Unit Delay13/1
  Sum15/1 -> MATLAB Function24/1(u)
  Demux10/5 -> Mux23/4
  Sum45/1 -> Scope74/1
  bdis53/1 -> Sum43/2
  Clock5/1 -> MATLAB Function25/2(t)
  MATLAB Function/1(y) -> Scope51/1, Scope85/2, Demux5/1
  [y_ma] -> Scope97/1
  MATLAB Function30/1(y) -> Demux14/1, Scope93/2, Scope71/1
  bdis51/1 -> Sum39/1
  Sum14/1 -> Unit Delay7/1
  [y_ma] -> Sum11/2, MATLAB Function13/2(ym)
  MATLAB Function29/1(y) -> Demux9/1, Scope92/2, Scope21/1
  Mux23/1 -> Sum26/1, MATLAB Function17/1(ya)
  Demux13/3 -> Mux15/3
  Sum21/1 -> Scope16/1
  Clock3/1 -> MATLAB Function/2(t)
  Unit Delay2/1 -> bdis21/1, adis2/1, Sum7/1
  Demux13/1 -> Mux15/1
  Clock6/1 -> MATLAB Function26/2(t)
  Demux7/3 -> Mux18/3
  [y_ma] -> Sum1/2, MATLAB Function8/2(ym)
  [V_vsi] -> bdis4/1, bdis3/1, bdis2/1
  [y_ma] -> Scope85/1
  Demux5/3 -> Mux16/3
  Sum28/1 -> Derivative8/1, Scope22/1
  Unit Delay9/1 -> bdis46/1, adis8/1, Sum34/1
  [y_ma] -> Scope90/1
  [V_vsi] -> bdis30/1, bdis29/1, bdis28/1
  [u_fs] -> bdis37/1
  Highpass Filter/1 -> Scope98/1
  Demux3/3 -> Mux13/3
  MATLAB Function25/1(y) -> Scope63/1, Scope88/2, Demux8/1
  Demux8/3 -> Mux19/3
  bdis8/1 -> Sum14/2
  bdis10/1 -> Sum16/1
  Demux7/2 -> Mux18/2
  [I3] -> bdis25/1, bdis24/1, bdis23/1
  MATLAB Function34/1(r) -> Scope107/1
  Demux14/3 -> Mux24/3
  Mux25/1 -> Sum40/1, MATLAB Function21/1(ya)
  Clock14/1 -> MATLAB Function37/2(t)
  Clock15/1 -> MATLAB Function34/2(t)
  [u_fs] -> bdis57/1
  connections:
  RL/LConn1 -- I sens A/RConn1 -- RL2/LConn1 -- RL1/LConn1
  Ground/LConn1 -- RL1/RConn1 -- RL2/RConn1 -- RL/RConn1
  1Ph_Inverter_bio/RConn2 -- Ground1/LConn1
  DC 1000V/LConn1 -- 1Ph_Inverter_bio/LConn2
  Rin/RConn1 -- 1Ph_Inverter_bio/LConn1
  1Ph_Inverter_diesel/RConn2 -- Ground3/LConn1
  1Ph_Inverter_diesel/RConn1 -- I sens A/LConn1 -- 1Ph_Inverter_bio/RConn1 -- 1Ph_Inverter_bio1/RConn1
  DC 1000V/RConn1 -- Rin/LConn1
  1Ph_Inverter_bio1/RConn2 -- Ground2/LConn1
  Subsystem/LConn1 -- 1Ph_Inverter_diesel/LConn1
  Subsystem/LConn2 -- 1Ph_Inverter_diesel/LConn2
  DIESEL + Rectifier System/LConn1 -- 1Ph_Inverter_bio1/LConn1
  DIESEL + Rectifier System/LConn2 -- 1Ph_Inverter_bio1/LConn2

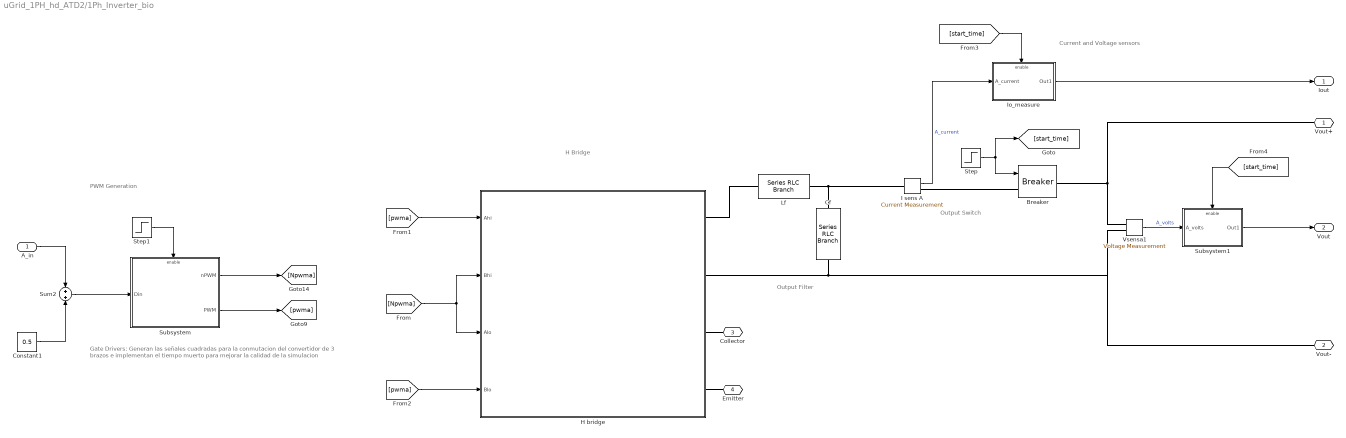
== system uGrid_1PH_hd_ATD2/1Ph_Inverter_bio ==
  note: PWM Generation
  note: H Bridge
  note: Output Filter
  note: Current and Voltage sensors
  note: Output Switch
  note: Gate Drivers: Generan las señales cuadradas para
      | la conmutacion del convertidor de 3 brazos e implementan el
      | tiempo muerto para mejorar la calidad de la simulacion
  A_in : Inport
  Breaker : powerlib/Elements/Breaker  InitialState=0  SwitchingTimes="[1/60  5/60]"  External=on  BreakerResistance=0.01  SnubberResistance=1e6  SnubberCapacitance=inf  Measurements=None  MoreParameters=on  NoBreakLoop=off
      settings: SourceProductName=Simscape Power Systems
  Cf : powerlib/Elements/Series RLC Branch  LConnTagsString=__new0  RConnTagsString=__new0  BranchType=C  Resistance=1  Inductance=1e-3  SetiL0=off  InitialCurrent=0  Capacitance=22e-6  Setx0=off  InitialVoltage=0  Measurements=None
  Constant1 : Constant  Value=0.5
  H bridge : Subsystem
      mask Display:
      | port_label('input', 1, '\fontsize{12} Ahi', 'texmode', 'on')
      | port_label('input', 2, '\fontsize{12} Alo', 'texmode', 'on')
      | port_label('input', 3, '\fontsize{12} Bhi', 'texmode', 'on')
      | port_label('input', 4, '\fontsize{12} Blo', 'texmode', 'on')
      | 
      | 
      | port_label('rconn', 1, '\fontsize{12} V_{out} +', 'texmode', 'on')
      | port_label('rconn', 2, '\fontsize{12} V_{out} -', 'texmode', 'on')
      | 
      | port_label('rconn', 3, '\fontsize{12} Collector', 'texmode', 'on')
      | port_label('rconn', 4, '\fontsize{12} Emitter', 'texmode', 'on')
      | 
      | lvx = [.1 .1];
      | lvy = [.1 .2];
      | lhx = [.1 .2];
      | lhy = [.1 .1];
      | 
      | 
      | % se dibujan los interruptores de la izquierda
      | plot(lvx+.07, lvy*.8+.028+.1)
      | plot(lvx+.1, lvy+.1)
      | plot(lhx*.5+.15, lhy+.1)
      | plot(lhx*.5+.15, lhy+.2)
      | plot(lhx*.5+.07, lhy+.15)
      | 
      | d=0.5;
      | 
      | plot(lvx+.07, lvy*.8+.028+.1+d)
      | plot(lvx+.1, lvy+.1+d)
      | plot(lhx*.5+.15, lhy+.1+d)
      | plot(lhx*.5+.15, lhy+.2+d)
      | plot(lhx*.5+.07, lhy+.15+d)
      | 
      | 
      | % se dibujan los interruptores del medio
      | h=.3;
      | 
      | %plot(lvx+.07+h, lvy*.8+.028+.1)
      | %plot(lvx+.1+h, lvy+.1)
      | %plot(lhx*.5+.15+h, lhy+.1)
      | %plot(lhx*.5+.15+h, lhy+.2)
      | %plot(lhx*.5+.07+h, lhy+.15)
      | 
      | %plot(lvx+.07+h, lvy*.8+.028+.1+d)
      | %plot(lvx+.1+h, lvy+.1+d)
      | %plot(lhx*.5+.15+h, lhy+.1+d)
      | %plot(lhx*.5+.15+h, lhy+.2+d)
      | %plot(lhx*.5+.07+h, lhy+.15+d)
      | 
      | % se dibujan los interruptores de la derecha
      | h=.6
      | 
      | plot(lvx+.07+h, lvy*.8+.028+.1)
      | plot(lvx+.1+h, lvy+.1)
      | plot(lhx*.5+.15+h, lhy+.1)
      | plot(lhx*.5+.15+h, lhy+.2)
      | plot(lhx*.5+.07+h, lhy+.15)
      | 
      | plot(lvx+.07+h, lvy*.8+.028+.1+d)
      | plot(lvx+.1+h, lvy+.1+d)
      | plot(lhx*.5+.15+h, lhy+.1+d)
      | plot(lhx*.5+.15+h, lhy+.2+d)
      | plot(lhx*.5+.07+h, lhy+.15+d)
      | 
      | 
      | % se conectan los interruptores.
      | plot(lvx+.15, lvy*4-.1)
      | %plot(lvx+.15+.3, lvy*4-.1)
      | plot(lvx+.15+.6, lvy*4-.1)
      | 
      | 
      | plot(lvx+.15, lvy+.7)
      | %plot(lvx+.15+.3, lvy+.7)
      | plot(lvx+.15+.6, lvy+.7)
      | 
      | plot(lvx+.15, lvy)
      | %plot(lvx+.15+.3, lvy)
      | plot(lvx+.15+.6, lvy)
      | 
      | plot(lhx*6-.35, lhy)
      | plot(lhx*6-.35, lhy+.8)
      | 
      | % raul esteban alzate 313 515 86 11
  I sens A : powerlib/Measurements/Current Measurement  PhasorSimulation=off  OutputType=Complex  PSBequivalent=0
  Io_measure : Subsystem
  Lf : powerlib/Elements/Series RLC Branch  LConnTagsString=__new0  RConnTagsString=__new0  BranchType=RL  Resistance=.1  Inductance=40e-3  SetiL0=off  InitialCurrent=0  Capacitance=1e-6  Setx0=off  InitialVoltage=0  Measurements=None
  Step : Step  Time=st_time  SampleTime=0
  Step1 : Step  Time=st_time  SampleTime=0
  Subsystem : Subsystem
  Subsystem1 : Subsystem
  Sum2 : Sum
  Vsensa1 : powerlib/Measurements/Voltage Measurement  PhasorSimulation=off  OutputType=Complex  PSBequivalent=0
  Vout+ : PMIOPort  Side=Right
  Vout- : PMIOPort  Port=2  Side=Right
  Collector : PMIOPort  Port=3  Side=Left
  Emitter : PMIOPort  Port=4  Side=Left
  Iout : Outport
  Vout : Outport  Port=2
  wires:
  Constant1/1 -> Sum2/2
  A_in/1 -> Sum2/1
  [pwma] -> H bridge/1(Ahi)
  [Npwma] -> H bridge/2(Bhi), H bridge/3(Alo)
  [pwma] -> H bridge/4(Blo)
  Step/1 -> [start_time], Breaker/1
  Sum2/1 -> Subsystem/1(Din)
  Subsystem/1(nPWM) -> [Npwma]
  Subsystem/2(PWM) -> [pwma]
  Step1/1 -> Subsystem/Enable
  I sens A/1 -> Io_measure/1(A_current)  "A_current"
  Io_measure/1(Out1) -> Iout/1
  [start_time] -> Io_measure/Enable
  Vsensa1/1 -> Subsystem1/1(A_volts)  "A_volts"
  Subsystem1/1(Out1) -> Vout/1
  [start_time] -> Subsystem1/Enable
  connections:
  H bridge/RConn3 -- Collector/RConn1
  H bridge/RConn4 -- Emitter/RConn1
  Lf/LConn1 -- H bridge/RConn1
  H bridge/RConn2 -- Vsensa1/LConn2 -- Vout-/RConn1 -- Cf/RConn1
  Breaker/LConn1 -- I sens A/RConn1
  Breaker/RConn1 -- Vout+/RConn1 -- Vsensa1/LConn1
  Cf/LConn1 -- I sens A/LConn1 -- Lf/RConn1

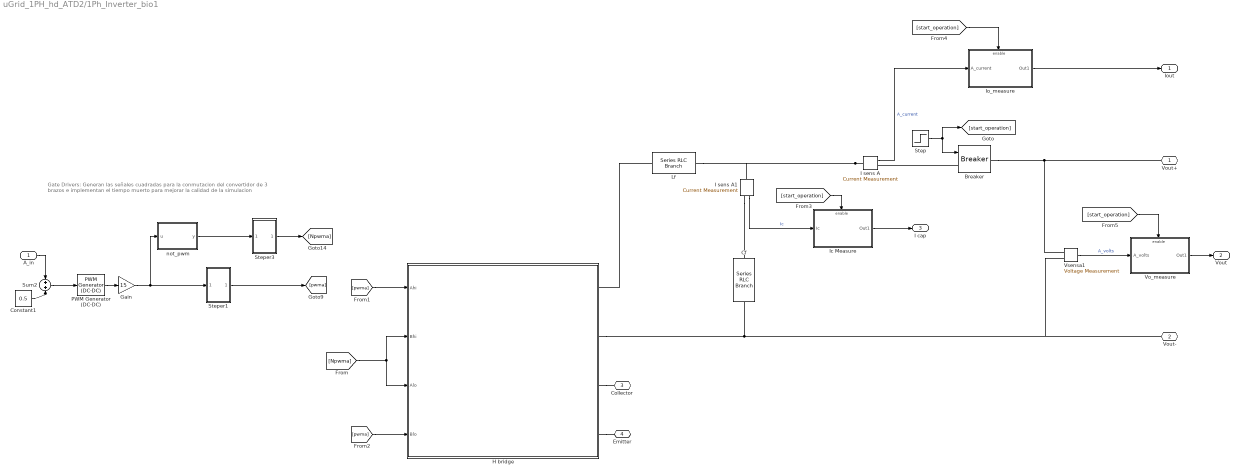
== system uGrid_1PH_hd_ATD2/1Ph_Inverter_bio1 ==
  note: Gate Drivers: Generan las señales cuadradas para
      | la conmutacion del convertidor de 3 brazos e implementan el
      | tiempo muerto para mejorar la calidad de la simulacion
  A_in : Inport
  Breaker : powerlib/Elements/Breaker  InitialState=0  SwitchingTimes="[1/60  5/60]"  External=on  BreakerResistance=0.01  SnubberResistance=1e6  SnubberCapacitance=inf  Measurements=None  MoreParameters=on  NoBreakLoop=off
      settings: SourceProductName=Simscape Power Systems
  Cf : powerlib/Elements/Series RLC Branch  LConnTagsString=__new0  RConnTagsString=__new0  BranchType=C  Resistance=1  Inductance=1e-3  SetiL0=off  InitialCurrent=0  Capacitance=610e-6  Setx0=off  InitialVoltage=0  Measurements=None
  Constant1 : Constant  Value=0.5
  Gain : Gain  Gain=15
  H bridge : Subsystem
      mask Display:
      | port_label('input', 1, '\fontsize{12} Ahi', 'texmode', 'on')
      | port_label('input', 2, '\fontsize{12} Alo', 'texmode', 'on')
      | port_label('input', 3, '\fontsize{12} Bhi', 'texmode', 'on')
      | port_label('input', 4, '\fontsize{12} Blo', 'texmode', 'on')
      | 
      | 
      | port_label('rconn', 1, '\fontsize{12} V_{out} +', 'texmode', 'on')
      | port_label('rconn', 2, '\fontsize{12} V_{out} -', 'texmode', 'on')
      | 
      | port_label('rconn', 3, '\fontsize{12} Collector', 'texmode', 'on')
      | port_label('rconn', 4, '\fontsize{12} Emitter', 'texmode', 'on')
      | 
      | lvx = [.1 .1];
      | lvy = [.1 .2];
      | lhx = [.1 .2];
      | lhy = [.1 .1];
      | 
      | 
      | % se dibujan los interruptores de la izquierda
      | plot(lvx+.07, lvy*.8+.028+.1)
      | plot(lvx+.1, lvy+.1)
      | plot(lhx*.5+.15, lhy+.1)
      | plot(lhx*.5+.15, lhy+.2)
      | plot(lhx*.5+.07, lhy+.15)
      | 
      | d=0.5;
      | 
      | plot(lvx+.07, lvy*.8+.028+.1+d)
      | plot(lvx+.1, lvy+.1+d)
      | plot(lhx*.5+.15, lhy+.1+d)
      | plot(lhx*.5+.15, lhy+.2+d)
      | plot(lhx*.5+.07, lhy+.15+d)
      | 
      | 
      | % se dibujan los interruptores del medio
      | h=.3;
      | 
      | %plot(lvx+.07+h, lvy*.8+.028+.1)
      | %plot(lvx+.1+h, lvy+.1)
      | %plot(lhx*.5+.15+h, lhy+.1)
      | %plot(lhx*.5+.15+h, lhy+.2)
      | %plot(lhx*.5+.07+h, lhy+.15)
      | 
      | %plot(lvx+.07+h, lvy*.8+.028+.1+d)
      | %plot(lvx+.1+h, lvy+.1+d)
      | %plot(lhx*.5+.15+h, lhy+.1+d)
      | %plot(lhx*.5+.15+h, lhy+.2+d)
      | %plot(lhx*.5+.07+h, lhy+.15+d)
      | 
      | % se dibujan los interruptores de la derecha
      | h=.6
      | 
      | plot(lvx+.07+h, lvy*.8+.028+.1)
      | plot(lvx+.1+h, lvy+.1)
      | plot(lhx*.5+.15+h, lhy+.1)
      | plot(lhx*.5+.15+h, lhy+.2)
      | plot(lhx*.5+.07+h, lhy+.15)
      | 
      | plot(lvx+.07+h, lvy*.8+.028+.1+d)
      | plot(lvx+.1+h, lvy+.1+d)
      | plot(lhx*.5+.15+h, lhy+.1+d)
      | plot(lhx*.5+.15+h, lhy+.2+d)
      | plot(lhx*.5+.07+h, lhy+.15+d)
      | 
      | 
      | % se conectan los interruptores.
      | plot(lvx+.15, lvy*4-.1)
      | %plot(lvx+.15+.3, lvy*4-.1)
      | plot(lvx+.15+.6, lvy*4-.1)
      | 
      | 
      | plot(lvx+.15, lvy+.7)
      | %plot(lvx+.15+.3, lvy+.7)
      | plot(lvx+.15+.6, lvy+.7)
      | 
      | plot(lvx+.15, lvy)
      | %plot(lvx+.15+.3, lvy)
      | plot(lvx+.15+.6, lvy)
      | 
      | plot(lhx*6-.35, lhy)
      | plot(lhx*6-.35, lhy+.8)
      | 
      | % raul esteban alzate 313 515 86 11
  I sens A : powerlib/Measurements/Current Measurement  PhasorSimulation=off  OutputType=Complex  PSBequivalent=0
  I sens A1 : powerlib/Measurements/Current Measurement  PhasorSimulation=off  OutputType=Complex  PSBequivalent=0
  Ic Measure : Subsystem
  Io_measure : Subsystem
  Lf : powerlib/Elements/Series RLC Branch  LConnTagsString=__new0  RConnTagsString=__new0  BranchType=RL  Resistance=1e-3  Inductance=5e-3  SetiL0=off  InitialCurrent=0  Capacitance=1e-6  Setx0=off  InitialVoltage=0  Measurements=None
  PWM Generator (DC-DC) : powerlib_meascontrol/Pulse & Signal Generators/PWM Generator (DC-DC)  Fsw=f_sw  Ts=samp_f
  Step : Step  Time=st_time  SampleTime=0
  Steper1 : Subsystem
  Steper3 : Subsystem
  Sum2 : Sum
  Vo_measure : Subsystem
  Vsensa1 : powerlib/Measurements/Voltage Measurement  PhasorSimulation=off  OutputType=Complex  PSBequivalent=0
  not_pwm : MATLAB Function  TreatAsAtomicUnit=on
  Vout+ : PMIOPort  Side=Right
  Vout- : PMIOPort  Port=2  Side=Right
  Collector : PMIOPort  Port=3  Side=Left
  Emitter : PMIOPort  Port=4  Side=Left
  Iout : Outport
  Vout : Outport  Port=2
  I cap : Outport  Port=3
  wires:
  not_pwm/1(y) -> Steper3/1(In1)
  Sum2/1 -> PWM Generator (DC-DC)/1
  PWM Generator (DC-DC)/1 -> Gain/1
  Constant1/1 -> Sum2/2
  A_in/1 -> Sum2/1
  Steper1/1(Out1) -> [pwma]
  Steper3/1(Out1) -> [Npwma]
  Gain/1 -> Steper1/1(In1), not_pwm/1(u)
  [pwma] -> H bridge/1(Ahi)
  [Npwma] -> H bridge/2(Bhi), H bridge/3(Alo)
  [pwma] -> H bridge/4(Blo)
  Step/1 -> [start_operation], Breaker/1
  I sens A1/1 -> Ic Measure/1(Ic)  "Ic"
  Ic Measure/1(Out1) -> I cap/1
  [start_operation] -> Ic Measure/Enable
  Vsensa1/1 -> Vo_measure/1(A_volts)  "A_volts"
  Vo_measure/1(Out1) -> Vout/1
  I sens A/1 -> Io_measure/1(A_current)  "A_current"
  Io_measure/1(Out1) -> Iout/1
  [start_operation] -> Io_measure/Enable
  [start_operation] -> Vo_measure/Enable
  connections:
  H bridge/RConn3 -- Collector/RConn1
  H bridge/RConn4 -- Emitter/RConn1
  Lf/LConn1 -- H bridge/RConn1
  H bridge/RConn2 -- Vout-/RConn1 -- Vsensa1/LConn2 -- Cf/RConn1
  Breaker/LConn1 -- I sens A/RConn1
  Breaker/RConn1 -- Vsensa1/LConn1 -- Vout+/RConn1
  I sens A/LConn1 -- Lf/RConn1 -- I sens A1/LConn1
  I sens A1/RConn1 -- Cf/LConn1
